simulink model "Ford_T3T6_ArchCnctnDigrm"  (R2016b)
settings: Solver=FixedStepDiscrete  StartTime=0.0  StopTime=10.0  RelTol=1e-3  EnableMultiTasking=on
libraries: canmsglib x15
(part 13 of 15)

== system Ford_T3T6_ArchCnctnDigrm/Vehicle Com/Rx Messages/Vehicle Data ==
  note: From COM
  note: From COM
  note: From COM
  note: From COM
  note: From COM
  Ford_SelDrvMdeChassis2_D_Rq : Ground
  Ignition_Status : Ground
  LifeCycMde_D_Actl : Ground
  MM054A_FordMsg083BusHiSpd : Subsystem  Tag=4.0.X  Description=The purpose of the Ford Message 083 Bus High Speed function is to provide the Electric Power Steering system with signal values for the Lane Detection Warning function from CAN. The Ford Message 083 function will perform the missing message diagnostics as well asprovide a validity flag for the signal values and received message. Detailed requirements have implemented the Ford DBC file for guidance.
      settings: AttributesFormatString=Version: %<Tag>
  MM072A_FordMsg3B3BusHiSpd : Subsystem  Tag=4.0.X  Description=The purpose of the Ford Message 3B3 Bus High Speed function is to provide the Electric PowerSteering system with signal values for the Trailer Back Up Assist and Electric Power Steering functions from CAN. The Ford Message 3B3 function will perform the missing message and signal invalid diagnostic as well as provide a validity signal for the received message.
      settings: AttributesFormatString=Version: %<Tag>
  MM076A_FordMsg40ABusHiSpd : Subsystem  Tag=4.0.X  Description=The purpose of the Ford Message 40A Bus High Speed function is to provide the Electric Power Steering systemwith signal values for the global configuration function from CAN.The Ford Message 40A function will perform the missing message.
      settings: AttributesFormatString=Version: %<Tag>
  MM079A_FordMsg41EBusHiSpd : Subsystem  Tag=4.0.X  Description="The purpose of the Ford Message 41E Bus High Speed function is to providethe Electric Power Steering system with signal values for the Select DriveMode  function from CAN. The Ford Message 41E function will perform themissing message and signal invalid diagnostics as well as provide a validity flag for the signal values and received message."
      settings: AttributesFormatString=Version: %<Tag>
  MM081A_FordMsg430BusHiSpd : Subsystem  Tag=4.0.X  Description=The purpose of the Ford Message 430 Bus High Speed function is to provide the Electric Power Steeringsystem with vehicle odometer, climate, and Trailer Back Up Assist signals from CAN. The Ford Message430 function will perform the missing message and signal invalid diagnostics as well as provide avalidity signal for the signal values and received message.
      settings: AttributesFormatString=Version: %<Tag>
  OdometerMasterValue : Ground
  TurnLghtSwtch_D_Stat : Ground
  VehicleGGCCData : Ground
  tag scope: ComIPduCallout_BodyInfo_3_FD1=global, ComIPduCallout_BrakeSysFeatures_3_FD1=global, ComIPduCallout_Cluster_Info1_FD1=global, ComIPduCallout_GGCC_Config_Mgmt_ID_1_FD1=global, ComIPduCallout_Steering_Data_FD1=global, ComTimeoutNotification_Ignition_Status=global, ComTimeoutNotification_OdometerMasterValue=global, ComTimeoutNotification_SelDrvMdeChassis2_D_Rq=global, ComTimeoutNotification_TurnLghtSwtch_D_Stat=global, ComTimeoutNotification_VehicleGGCCData=global, FordVehGlbRealTi=global, FordVehIdnNr=global, FordVehIgnSts=global, FordVehIgnStsVld=global, FordVehLifeCycMod=global, FordVehOdom=global, FordVehPenSelDrvMod=global, FordVehSelDrvModChassisVld=global, FordVehTireCircum=global, FordVehTurnSigSwtStsRaw=global, FordVehTurnSigVld=global
  wires:
  [ClrDiagcFlgProxy] -> MM054A_FordMsg083BusHiSpd/1(ClrDiagcFlgProxy)
  [FordCanDtcInhb] -> MM054A_FordMsg083BusHiSpd/2(FordCanDtcInhb)
  [FordEpsLifeCycMod] -> MM054A_FordMsg083BusHiSpd/3(FordEpsLifeCycMod)
  [LaneDetnWarnEnad] -> MM054A_FordMsg083BusHiSpd/4(FordLaneDetnWarnEnad)
  TurnLghtSwtch_D_Stat/1 -> MM054A_FordMsg083BusHiSpd/5(Ford_TurnLghtSwtch_D_Stat1)
  [GetRefTmr100MicroSec32bit] -> MM054A_FordMsg083BusHiSpd/6(GetRefTmr100MicroSec32bit)
  [GetTiSpan100MicroSec32bit] -> MM054A_FordMsg083BusHiSpd/7(GetTiSpan100MicroSec32bit)
  [SetNtcSts] -> MM054A_FordMsg083BusHiSpd/8(SetNtcSts)
  MM054A_FordMsg083BusHiSpd/1(FordVehTurnSigSwtStsRaw) -> [FordVehTurnSigSwtStsRaw]
  MM054A_FordMsg083BusHiSpd/2(FordVehTurnSigVld) -> [FordVehTurnSigVld]
  MM054A_FordMsg083BusHiSpd/3(ComIPduCallout_Steering_Data_FD1) -> [ComIPduCallout_Steering_Data_FD1]
  MM054A_FordMsg083BusHiSpd/4(ComTimeoutNotification_TurnLghtSwtch_D_Stat) -> [ComTimeoutNotification_TurnLghtSwtch_D_Stat]
  [ClrDiagcFlgProxy] -> MM072A_FordMsg3B3BusHiSpd/1(ClrDiagcFlgProxy)
  [FordCanDtcInhb] -> MM072A_FordMsg3B3BusHiSpd/2(FordCanDtcInhb)
  [FordEpsLifeCycMod] -> MM072A_FordMsg3B3BusHiSpd/3(FordEpsLifeCycMod)
  Ignition_Status/1 -> MM072A_FordMsg3B3BusHiSpd/4(Ford_Ignition_Status1)
  LifeCycMde_D_Actl/1 -> MM072A_FordMsg3B3BusHiSpd/5(Ford_LifeCycMde_D_Actl1)
  [GetRefTmr100MicroSec32bit] -> MM072A_FordMsg3B3BusHiSpd/6(GetRefTmr100MicroSec32bit)
  [GetTiSpan100MicroSec32bit] -> MM072A_FordMsg3B3BusHiSpd/7(GetTiSpan100MicroSec32bit)
  [SetNtcSts] -> MM072A_FordMsg3B3BusHiSpd/8(SetNtcSts)
  MM072A_FordMsg3B3BusHiSpd/1(FordVehIgnSts) -> [FordVehIgnSts]
  MM072A_FordMsg3B3BusHiSpd/2(FordVehIgnStsVld) -> [FordVehIgnStsVld]
  MM072A_FordMsg3B3BusHiSpd/3(FordVehLifeCycMod) -> [FordVehLifeCycMod]
  MM072A_FordMsg3B3BusHiSpd/4(ComIPduCallout_BodyInfo_3_FD1) -> [ComIPduCallout_BodyInfo_3_FD1]
  MM072A_FordMsg3B3BusHiSpd/5(ComTimeoutNotification_Ignition_Status) -> [ComTimeoutNotification_Ignition_Status]
  [ClrDiagcFlgProxy] -> MM076A_FordMsg40ABusHiSpd/1(ClrDiagcFlgProxy)
  [FordCanDtcInhb] -> MM076A_FordMsg40ABusHiSpd/2(FordCanDtcInhb)
  [FordEpsLifeCycMod] -> MM076A_FordMsg40ABusHiSpd/3(FordEpsLifeCycMod)
  VehicleGGCCData/1 -> MM076A_FordMsg40ABusHiSpd/4(Ford_VehicleGGCCData)
  [GetRefTmr100MicroSec32bit] -> MM076A_FordMsg40ABusHiSpd/5(GetRefTmr100MicroSec32bit)
  [GetTiSpan100MicroSec32bit] -> MM076A_FordMsg40ABusHiSpd/6(GetTiSpan100MicroSec32bit)
  [SetNtcSts] -> MM076A_FordMsg40ABusHiSpd/7(SetNtcSts)
  MM076A_FordMsg40ABusHiSpd/1(FordVehGlbRealTi) -> [FordVehGlbRealTi]
  MM076A_FordMsg40ABusHiSpd/2(FordVehIdnNr) -> [FordVehIdnNr]
  MM076A_FordMsg40ABusHiSpd/3(FordVehTireCircum) -> [FordVehTireCircum]
  MM076A_FordMsg40ABusHiSpd/4(ComIPduCallout_GGCC_Config_Mgmt_ID_1_FD1) -> [ComIPduCallout_GGCC_Config_Mgmt_ID_1_FD1]
  MM076A_FordMsg40ABusHiSpd/5(ComTimeoutNotification_VehicleGGCCData) -> [ComTimeoutNotification_VehicleGGCCData]
  [ClrDiagcFlgProxy] -> MM081A_FordMsg430BusHiSpd/1(ClrDiagcFlgProxy)
  [FordCanDtcInhb] -> MM081A_FordMsg430BusHiSpd/2(FordCanDtcInhb)
  [FordEpsLifeCycMod] -> MM081A_FordMsg430BusHiSpd/3(FordEpsLifeCycMod)
  OdometerMasterValue/1 -> MM081A_FordMsg430BusHiSpd/4(Ford_OdometerMasterValue)
  [GetRefTmr100MicroSec32bit] -> MM081A_FordMsg430BusHiSpd/5(GetRefTmr100MicroSec32bit)
  [GetTiSpan100MicroSec32bit] -> MM081A_FordMsg430BusHiSpd/6(GetTiSpan100MicroSec32bit)
  [SetNtcSts] -> MM081A_FordMsg430BusHiSpd/7(SetNtcSts)
  MM081A_FordMsg430BusHiSpd/1(FordVehOdom) -> [FordVehOdom]
  MM081A_FordMsg430BusHiSpd/2(ComIPduCallout_Cluster_Info1_FD1) -> [ComIPduCallout_Cluster_Info1_FD1]
  MM081A_FordMsg430BusHiSpd/3(ComTimeoutNotification_OdometerMasterValue) -> [ComTimeoutNotification_OdometerMasterValue]
  [ClrDiagcFlgProxy] -> MM079A_FordMsg41EBusHiSpd/1(ClrDiagcFlgProxy)
  [FordCanDtcInhb] -> MM079A_FordMsg41EBusHiSpd/2(FordCanDtcInhb)
  [FordEpsLifeCycMod] -> MM079A_FordMsg41EBusHiSpd/3(FordEpsLifeCycMod)
  [FordSelDrvModEnad] -> MM079A_FordMsg41EBusHiSpd/4(FordSelDrvModEnad)
  Ford_SelDrvMdeChassis2_D_Rq/1 -> MM079A_FordMsg41EBusHiSpd/5(Ford_SelDrvMdeChassis2_D_Rq1)
  [GetRefTmr100MicroSec32bit] -> MM079A_FordMsg41EBusHiSpd/6(GetRefTmr100MicroSec32bit)
  [GetTiSpan100MicroSec32bit] -> MM079A_FordMsg41EBusHiSpd/7(GetTiSpan100MicroSec32bit)
  [SetNtcSts] -> MM079A_FordMsg41EBusHiSpd/8(SetNtcSts)
  MM079A_FordMsg41EBusHiSpd/1(FordVehPenSelDrvMod) -> [FordVehPenSelDrvMod]
  MM079A_FordMsg41EBusHiSpd/2(FordVehSelDrvModChassisVld) -> [FordVehSelDrvModChassisVld]
  MM079A_FordMsg41EBusHiSpd/3(ComIPduCallout_BrakeSysFeatures_3_FD1) -> [ComIPduCallout_BrakeSysFeatures_3_FD1]
  MM079A_FordMsg41EBusHiSpd/4(ComTimeoutNotification_SelDrvMdeChassis2_D_Rq) -> [ComTimeoutNotification_SelDrvMdeChassis2_D_Rq]

== system Ford_T3T6_ArchCnctnDigrm/Vehicle Com/Rx Messages/Wheel Data ==
  note: From COM
  note: From COM
  note: From COM
  note: From COM
  ElPw_D_Stat : Ground
  ElPw_D_StatStrtStop : Ground
  Ground : Ground
  MM055A_FordMsg08ABusHiSpd : Subsystem  Tag=4.0.X  Description=The purpose of the Ford Message 08A Bus High Speed function is to provide the Electric Power Steering system with signal values for the EAC feature. The Ford Message 08A function will perform the missing message and signal invalid diagnostics
      settings: AttributesFormatString=Version: %<Tag>
  MM059A_FordMsg167BusHiSpd : Subsystem  Tag=2.0.0  Description=The purpose of the Ford Message 0167 Bus HighSpeed function is to provide the EPS system with signal valuesfor the System State, Voltage Diagnostic, Start Stop, and TorqueSteer Compensation functions from CAN. The Ford Message 167 functionwill perform the missing message and signal invalid diagnostics aswell as provide a validity flag for the signal valuesand received message.
      settings: AttributesFormatString=Version: %<Tag>
  MM064A_FordMsg216BusHiSpd : Subsystem  Tag=4.0.X  Description=The purpose of the Ford Message 216 Bus High Speedfunction is to provide the Electric Power Steering system with signalvalues for the Trailer Back Up Assist, Torque Steer Compensation,and Brake Oscillation Reduction functions from CAN. The Ford Message216 function will perform the missing message diagnostic as wellas provide a validity signal for the received message.
      settings: AttributesFormatString=Version: %<Tag>
  MM065A_FordMsg217BusHiSpd : Subsystem  Tag=4.0.X  Description=The purpose of the Ford Message 217 Bus High Speed function is to providethe Electric Power Steering system with signal values for vehicle speed, Active Nibble Control,TSC, Brake Oscillation Reduction, and Trailer Back Up Assist functions from CAN. The Ford Message 217Bus High Speed function will perform the missing message and signal invalid diagnostics as well as providea validity signal for the signal values and received message.
      settings: AttributesFormatString=Version: %<Tag>
  PrplWhlTot2_Tq_Actl : Ground
  PwPckTq_D_Stat : Ground
  SteWhlRelCalib_An_Sns1 : Ground
  WhlFl_W_Meas1 : Ground
  WhlFr_W_Meas1 : Ground
  WhlRl_W_Meas1 : Ground
  WhlRr_W_Meas1 : Ground
  tag scope: ComIPduCallout_ActiveFrontSteering_Stat2_FD1=global, ComIPduCallout_VehicleOperatingModes_HS2=global, ComIPduCallout_WheelData_FD1=global, ComIPduCallout_WheelSpeed_FD1=global, ComTimeoutNotification_PwPckTq_D_Stat=global, ComTimeoutNotification_SteWhlRelCalib_An_Sns=global, ComTimeoutNotification_WhlDirFl_D_Actl=global, ComTimeoutNotification_WhlFl_W_Meas=global, FordActvFrntSteerModlSteerWhlAgVldInt=global, FordVehActvFrntSteerModlSteerWhlAg=global, FordVehActvFrntSteerModlSteerWhlAgRaw=global, FordVehElecPwrStrtStopSts=global, FordVehElecPwrSts=global, FordVehFrntLeWhlCntrDirVld=global, FordVehFrntLeWhlDirRaw=global, FordVehFrntLeWhlRollgCntr=global, FordVehFrntLeWhlSpd=global, FordVehFrntLeWhlSpdRaw=global, FordVehFrntLeWhlSpdVld=global, FordVehFrntRiWhlCntrDirVld=global, FordVehFrntRiWhlDirRaw=global, FordVehFrntRiWhlRollgCntr=global, FordVehFrntRiWhlSpd=global, FordVehFrntRiWhlSpdRaw=global, FordVehFrntRiWhlSpdVld=global, FordVehPrpnWhlTq=global, FordVehPrpnWhlTqRaw=global, FordVehPrpnWhlTqVld=global, FordVehPwrpkTqSts=global, FordVehReLeWhlCntrDirVld=global, FordVehReLeWhlDirRaw=global, FordVehReLeWhlRollgCntr=global, FordVehReLeWhlSpd=global, FordVehReLeWhlSpdRaw=global, FordVehReLeWhlSpdVld=global, FordVehReRiWhlCntrDirVld=global, FordVehReRiWhlDirRaw=global, FordVehReRiWhlRollgCntr=global, FordVehReRiWhlSpd=global, FordVehReRiWhlSpdRaw=global, FordVehReRiWhlSpdVld=global
  wires:
  [ClrDiagcFlgProxy] -> MM059A_FordMsg167BusHiSpd/1(ClrDiagcFlgProxy)
  [FordBrkOscnRednEnad] -> MM059A_FordMsg167BusHiSpd/2(FordBrkOscnRednEnad)
  [FordCanDtcInhb] -> MM059A_FordMsg167BusHiSpd/3(FordCanDtcInhb)
  [FordEpsLifeCycMod] -> MM059A_FordMsg167BusHiSpd/4(FordEpsLifeCycMod)
  [FordInvldMsgDiagcInhb] -> MM059A_FordMsg167BusHiSpd/5(FordInvldMsgDiagcInhb)
  [FordMfgDiagcInhb] -> MM059A_FordMsg167BusHiSpd/6(FordMfgDiagcInhb)
  [FordMissMsgDiagcInhb] -> MM059A_FordMsg167BusHiSpd/7(FordMissMsgDiagcInhb)
  [FordTqSteerCmpEnad] -> MM059A_FordMsg167BusHiSpd/8(FordTqSteerCmpEnad)
  [FordTrlrBackupAssiEnad] -> MM059A_FordMsg167BusHiSpd/9(FordTrlrBackUpAssiEnad)
  ElPw_D_Stat/1 -> MM059A_FordMsg167BusHiSpd/10(Ford_ElPw_D_Stat1)
  [GetRefTmr100MicroSec32bit] -> MM059A_FordMsg167BusHiSpd/14(GetRefTmr100MicroSec32bit)
  [GetTiSpan100MicroSec32bit] -> MM059A_FordMsg167BusHiSpd/15(GetTiSpan100MicroSec32bit)
  [SetNtcSts] -> MM059A_FordMsg167BusHiSpd/16(SetNtcSts)
  MM059A_FordMsg167BusHiSpd/1(FordVehElecPwrStrtStopSts) -> [FordVehElecPwrStrtStopSts]
  MM059A_FordMsg167BusHiSpd/2(FordVehElecPwrSts) -> [FordVehElecPwrSts]
  MM059A_FordMsg167BusHiSpd/3(FordVehPrpnWhlTq) -> [FordVehPrpnWhlTq]
  MM059A_FordMsg167BusHiSpd/4(FordVehPrpnWhlTqRaw) -> [FordVehPrpnWhlTqRaw]
  MM059A_FordMsg167BusHiSpd/5(FordVehPrpnWhlTqVld) -> [FordVehPrpnWhlTqVld]
  MM059A_FordMsg167BusHiSpd/6(FordVehPwrpkTqSts) -> [FordVehPwrpkTqSts]
  MM059A_FordMsg167BusHiSpd/7(ComIPduCallout_VehicleOperatingModes_HS2) -> [ComIPduCallout_VehicleOperatingModes_HS2]
  MM059A_FordMsg167BusHiSpd/8(ComTimeoutNotification_PwPckTq_D_Stat) -> [ComTimeoutNotification_PwPckTq_D_Stat]
  ElPw_D_StatStrtStop/1 -> MM059A_FordMsg167BusHiSpd/11(Ford_ElPw_D_StatStrtStop1)
  PrplWhlTot2_Tq_Actl/1 -> MM059A_FordMsg167BusHiSpd/12(Ford_PrplWhlTot2_Tq_Actl)
  PwPckTq_D_Stat/1 -> MM059A_FordMsg167BusHiSpd/13(Ford_PwPckTq_D_Stat1)
  [ClrDiagcFlgProxy] -> MM065A_FordMsg217BusHiSpd/1(ClrDiagcFlgProxy)
  [FordAbsPrsnt] -> MM065A_FordMsg217BusHiSpd/2(FordAbsPrsnt)
  [FordActvNiblCtrlEnad] -> MM065A_FordMsg217BusHiSpd/3(FordActvNiblCtrlEnad)
  [FordBrkOscnRednEnad] -> MM065A_FordMsg217BusHiSpd/4(FordBrkOscnRednEnad)
  [FordCanDtcInhb] -> MM065A_FordMsg217BusHiSpd/5(FordCanDtcInhb)
  [FordEpsLifeCycMod] -> MM065A_FordMsg217BusHiSpd/6(FordEpsLifeCycMod)
  [FordTqSteerCmpEnad] -> MM065A_FordMsg217BusHiSpd/7(FordTqSteerCmpEnad)
  [FordTrlrBackupAssiEnad] -> MM065A_FordMsg217BusHiSpd/8(FordTrlrBackupAssiEnad)
  [GetRefTmr100MicroSec32bit] -> MM065A_FordMsg217BusHiSpd/13(GetRefTmr100MicroSec32bit)
  [GetTiSpan100MicroSec32bit] -> MM065A_FordMsg217BusHiSpd/14(GetTiSpan100MicroSec32bit)
  [SetNtcSts] -> MM065A_FordMsg217BusHiSpd/15(SetNtcSts)
  MM065A_FordMsg217BusHiSpd/1(FordVehFrntLeWhlSpd) -> [FordVehFrntLeWhlSpd]
  MM065A_FordMsg217BusHiSpd/2(FordVehFrntLeWhlSpdRaw) -> [FordVehFrntLeWhlSpdRaw]
  MM065A_FordMsg217BusHiSpd/3(FordVehFrntLeWhlSpdVld) -> [FordVehFrntLeWhlSpdVld]
  MM065A_FordMsg217BusHiSpd/4(FordVehFrntRiWhlSpd) -> [FordVehFrntRiWhlSpd]
  MM065A_FordMsg217BusHiSpd/5(FordVehFrntRiWhlSpdRaw) -> [FordVehFrntRiWhlSpdRaw]
  MM065A_FordMsg217BusHiSpd/6(FordVehFrntRiWhlSpdVld) -> [FordVehFrntRiWhlSpdVld]
  MM065A_FordMsg217BusHiSpd/7(FordVehReLeWhlSpd) -> [FordVehReLeWhlSpd]
  MM065A_FordMsg217BusHiSpd/8(FordVehReLeWhlSpdRaw) -> [FordVehReLeWhlSpdRaw]
  MM065A_FordMsg217BusHiSpd/9(FordVehReLeWhlSpdVld) -> [FordVehReLeWhlSpdVld]
  MM065A_FordMsg217BusHiSpd/10(FordVehReRiWhlSpd) -> [FordVehReRiWhlSpd]
  MM065A_FordMsg217BusHiSpd/11(FordVehReRiWhlSpdRaw) -> [FordVehReRiWhlSpdRaw]
  MM065A_FordMsg217BusHiSpd/12(FordVehReRiWhlSpdVld) -> [FordVehReRiWhlSpdVld]
  MM065A_FordMsg217BusHiSpd/13(ComIPduCallout_WheelSpeed_FD1) -> [ComIPduCallout_WheelSpeed_FD1]
  MM065A_FordMsg217BusHiSpd/14(ComTimeoutNotification_WhlFl_W_Meas) -> [ComTimeoutNotification_WhlFl_W_Meas]
  WhlFl_W_Meas1/1 -> MM065A_FordMsg217BusHiSpd/9(Ford_WhlFl_W_Meas)
  WhlFr_W_Meas1/1 -> MM065A_FordMsg217BusHiSpd/10(Ford_WhlFr_W_Meas)
  WhlRl_W_Meas1/1 -> MM065A_FordMsg217BusHiSpd/11(Ford_WhlRl_W_Meas)
  WhlRr_W_Meas1/1 -> MM065A_FordMsg217BusHiSpd/12(Ford_WhlRr_W_Meas)
  [ClrDiagcFlgProxy] -> MM064A_FordMsg216BusHiSpd/1(ClrDiagcFlgProxy)
  [FordBrkOscnRednEnad] -> MM064A_FordMsg216BusHiSpd/2(FordBrkOscnRednEnad)
  [FordCanDtcInhb] -> MM064A_FordMsg216BusHiSpd/3(FordCanDtcInhb)
  [FordEpsLifeCycMod] -> MM064A_FordMsg216BusHiSpd/4(FordEpsLifeCycMod)
  [FordMfgDiagcInhb] -> MM064A_FordMsg216BusHiSpd/5(FordMfgDiagcInhb)
  [FordMissMsgDiagcInhb] -> MM064A_FordMsg216BusHiSpd/6(FordMissMsgDiagcInhb)
  [FordTqSteerCmpEnad] -> MM064A_FordMsg216BusHiSpd/7(FordTqSteerCmpEnad)
  [FordTrlrBackupAssiEnad] -> MM064A_FordMsg216BusHiSpd/8(FordTrlrBackUpAssiEnad)
  Ground/1 -> MM064A_FordMsg216BusHiSpd/16(Ford_WhlRotatRr_No_Cnt), MM064A_FordMsg216BusHiSpd/15(Ford_WhlRotatRl_No_Cnt), MM064A_FordMsg216BusHiSpd/14(Ford_WhlRotatFr_No_Cnt), MM064A_FordMsg216BusHiSpd/13(Ford_WhlRotatFl_No_Cnt), MM064A_FordMsg216BusHiSpd/12(Ford_WhlDirRr_D_Actl1), MM064A_FordMsg216BusHiSpd/11(Ford_WhlDirRl_D_Actl1), MM064A_FordMsg216BusHiSpd/10(Ford_WhlDirFr_D_Actl1), MM064A_FordMsg216BusHiSpd/9(Ford_WhlDirFl_D_Actl1)
  [GetRefTmr100MicroSec32bit] -> MM064A_FordMsg216BusHiSpd/17(GetRefTmr100MicroSec32bit)
  [GetTiSpan100MicroSec32bit] -> MM064A_FordMsg216BusHiSpd/18(GetTiSpan100MicroSec32bit)
  [SetNtcSts] -> MM064A_FordMsg216BusHiSpd/19(SetNtcSts)
  MM064A_FordMsg216BusHiSpd/1(FordVehFrntLeWhlCntrDirVld) -> [FordVehFrntLeWhlCntrDirVld]
  MM064A_FordMsg216BusHiSpd/2(FordVehFrntLeWhlDirRaw) -> [FordVehFrntLeWhlDirRaw]
  MM064A_FordMsg216BusHiSpd/3(FordVehFrntLeWhlRollgCntr) -> [FordVehFrntLeWhlRollgCntr]
  MM064A_FordMsg216BusHiSpd/4(FordVehFrntRiWhlCntrDirVld) -> [FordVehFrntRiWhlCntrDirVld]
  MM064A_FordMsg216BusHiSpd/5(FordVehFrntRiWhlDirRaw) -> [FordVehFrntRiWhlDirRaw]
  MM064A_FordMsg216BusHiSpd/6(FordVehFrntRiWhlRollgCntr) -> [FordVehFrntRiWhlRollgCntr]
  MM064A_FordMsg216BusHiSpd/7(FordVehReLeWhlCntrDirVld) -> [FordVehReLeWhlCntrDirVld]
  MM064A_FordMsg216BusHiSpd/8(FordVehReLeWhlDirRaw) -> [FordVehReLeWhlDirRaw]
  MM064A_FordMsg216BusHiSpd/9(FordVehReLeWhlRollgCntr) -> [FordVehReLeWhlRollgCntr]
  MM064A_FordMsg216BusHiSpd/10(FordVehReRiWhlCntrDirVld) -> [FordVehReRiWhlCntrDirVld]
  MM064A_FordMsg216BusHiSpd/11(FordVehReRiWhlDirRaw) -> [FordVehReRiWhlDirRaw]
  MM064A_FordMsg216BusHiSpd/12(FordVehReRiWhlRollgCntr) -> [FordVehReRiWhlRollgCntr]
  MM064A_FordMsg216BusHiSpd/13(ComIPduCallout_WheelData_FD1) -> [ComIPduCallout_WheelData_FD1]
  MM064A_FordMsg216BusHiSpd/14(ComTimeoutNotification_WhlDirFl_D_Actl) -> [ComTimeoutNotification_WhlDirFl_D_Actl]
  [ClrDiagcFlgProxy] -> MM055A_FordMsg08ABusHiSpd/1(ClrDiagcFlgProxy)
  [ActvFrntSteerPrsnt] -> MM055A_FordMsg08ABusHiSpd/2(FordActvFrntSteerPrsnt)
  [FordCanDtcInhb] -> MM055A_FordMsg08ABusHiSpd/3(FordCanDtcInhb)
  [FordEpsLifeCycMod] -> MM055A_FordMsg08ABusHiSpd/4(FordEpsLifeCycMod)
  SteWhlRelCalib_An_Sns1/1 -> MM055A_FordMsg08ABusHiSpd/5(Ford_SteWhlRelCalib_An_Sns)
  [GetRefTmr100MicroSec32bit] -> MM055A_FordMsg08ABusHiSpd/6(GetRefTmr100MicroSec32bit)
  [GetTiSpan100MicroSec32bit] -> MM055A_FordMsg08ABusHiSpd/7(GetTiSpan100MicroSec32bit)
  [SetNtcSts] -> MM055A_FordMsg08ABusHiSpd/8(SetNtcSts)
  MM055A_FordMsg08ABusHiSpd/1(FordActvFrntSteerModlSteerWhlAgVldInt) -> [FordActvFrntSteerModlSteerWhlAgVldInt]
  MM055A_FordMsg08ABusHiSpd/2(FordVehActvFrntSteerModlSteerWhlAg) -> [FordVehActvFrntSteerModlSteerWhlAg]
  MM055A_FordMsg08ABusHiSpd/3(FordVehActvFrntSteerModlSteerWhlAgRaw) -> [FordVehActvFrntSteerModlSteerWhlAgRaw]
  MM055A_FordMsg08ABusHiSpd/4(ComIPduCallout_ActiveFrontSteering_Stat2_FD1) -> [ComIPduCallout_ActiveFrontSteering_Stat2_FD1]
  MM055A_FordMsg08ABusHiSpd/5(ComTimeoutNotification_SteWhlRelCalib_An_Sns) -> [ComTimeoutNotification_SteWhlRelCalib_An_Sns]

== system Ford_T3T6_ArchCnctnDigrm/Vehicle Com/Rx Messages/Yaw Rate ==
  note: From COM
  note: From COM
  note: From COM
  Ford_TrlrSnsId_No_Act : Ground
  MM056A_FordMsg091BusHiSpd : Subsystem  Tag=0.0.X
      settings: AttributesFormatString=Version: %<Tag>
  MM082A_FordMsg452BusHiSpd : Subsystem  Tag=1.0.X  Description=The purpose of the Ford Message 452 Bus High Speed function is to provide the Electric Power Steering system with Trailer Back up Assist and Gear Lever Position signals from CAN. The Ford Message 452 function will perform the missing message and signal invalid diagnostics as well as provide a validity signal for the signal values and received message.
      settings: AttributesFormatString=Version: %<Tag>
  MM089A_FordMsg4B0BusHiSpd : Subsystem  Tag=4.0.X  Description=The purpose of the Ford Message 4B0 Bus High Speed function is to provide the Electric Power Steering system with signal values for the Torque Steer Compensation, Brake Oscillation Reduction, Lane Detection Warning, LKA, Traffic Jam Assist, Lane Center Assist, and Evasive Steer Assist functions from CAN. The Ford Message 4B0 function will perform the missing message and signal invalid diagnostics as well as provide a validity flag for the signal values and received message.
      settings: AttributesFormatString=Version: %<Tag>
  VehYaw_W_Actl : Ground
  YawStabilityIndex : Ground
  tag scope: ComIPduCallout_ABS_BrkBst_Data_FD1=global, ComIPduCallout_TrailerAid_Stat1_FD1=global, ComIPduCallout_Yaw_Data_FD1=global, ComTimeoutNotification_TrlrSnsId_No_Actl=global, ComTimeoutNotification_VehYaw_W_Actl=global, ComTimeoutNotification_YawStabilityIndex=global, FordVehYawRate=global, FordVehYawRateRaw=global, FordVehYawRateRawVld=global, FordVehYawRateSnsrIdyHi=global, FordVehYawRateSnsrIdyLo=global, FordVehYawStabyRaw=global, FordVehYawStabyVld=global
  wires:
  [ClrDiagcFlgProxy] -> MM056A_FordMsg091BusHiSpd/1(ClrDiagcFlgProxy)
  [FordCanDtcInhb] -> MM056A_FordMsg091BusHiSpd/2(FordCanDtcInhb)
  [FordEpsLifeCycMod] -> MM056A_FordMsg091BusHiSpd/3(FordEpsLifeCycMod)
  [FordInvldMsgDiagcInhb] -> MM056A_FordMsg091BusHiSpd/4(FordInvldMsgDiagcInhb)
  [FordMfgDiagcInhb] -> MM056A_FordMsg091BusHiSpd/5(FordMfgDiagcInhb)
  [FordMissMsgDiagcInhb] -> MM056A_FordMsg091BusHiSpd/6(FordMissMsgDiagcInhb)
  [FordTrlrBackupAssiEnad] -> MM056A_FordMsg091BusHiSpd/7(FordTrlrBackupAssiEnad)
  VehYaw_W_Actl/1 -> MM056A_FordMsg091BusHiSpd/8(Ford_VehYaw_W_Actl)
  [FordLaneCentrAssiEnad] -> MM056A_FordMsg091BusHiSpd/9(FordLaneCentrAssiEnad)
  [FordTrfcJamAssiEnad] -> MM056A_FordMsg091BusHiSpd/10(FordTrfcJamAssiEnad)
  [GetRefTmr100MicroSec32bit] -> MM056A_FordMsg091BusHiSpd/11(GetRefTmr100MicroSec32bit)
  [GetTiSpan100MicroSec32bit] -> MM056A_FordMsg091BusHiSpd/12(GetTiSpan100MicroSec32bit)
  [SetNtcSts] -> MM056A_FordMsg091BusHiSpd/13(SetNtcSts)
  MM056A_FordMsg091BusHiSpd/1(FordVehYawRate) -> [FordVehYawRate]
  MM056A_FordMsg091BusHiSpd/2(FordVehYawRateRaw) -> [FordVehYawRateRaw]
  MM056A_FordMsg091BusHiSpd/3(FordVehYawRateRawVld) -> [FordVehYawRateRawVld]
  MM056A_FordMsg091BusHiSpd/4(ComIPduCallout_Yaw_Data_FD1) -> [ComIPduCallout_Yaw_Data_FD1]
  MM056A_FordMsg091BusHiSpd/5(ComTimeoutNotification_VehYaw_W_Actl) -> [ComTimeoutNotification_VehYaw_W_Actl]
  [ClrDiagcFlgProxy] -> MM082A_FordMsg452BusHiSpd/1(ClrDiagcFlgProxy)
  [FordCanDtcInhb] -> MM082A_FordMsg452BusHiSpd/2(FordCanDtcInhb)
  [FordEpsLifeCycMod] -> MM082A_FordMsg452BusHiSpd/3(FordEpsLifeCycMod)
  [FordInvldMsgDiagcInhb] -> MM082A_FordMsg452BusHiSpd/4(FordInvldMsgDiagcInhb)
  [FordMfgDiagcInhb] -> MM082A_FordMsg452BusHiSpd/5(FordMfgDiagcInhb)
  [FordMissMsgDiagcInhb] -> MM082A_FordMsg452BusHiSpd/6(FordMissMsgDiagcInhb)
  [FordTrlrBackupAssiEnad] -> MM082A_FordMsg452BusHiSpd/7(FordTrlrBackupAssiEnad)
  Ford_TrlrSnsId_No_Act/1 -> MM082A_FordMsg452BusHiSpd/8(Ford_TrlrSnsId_No_Act)
  [GetRefTmr100MicroSec32bit] -> MM082A_FordMsg452BusHiSpd/9(GetRefTmr100MicroSec32bit)
  [GetTiSpan100MicroSec32bit] -> MM082A_FordMsg452BusHiSpd/10(GetTiSpan100MicroSec32bit)
  [SetNtcSts] -> MM082A_FordMsg452BusHiSpd/11(SetNtcSts)
  MM082A_FordMsg452BusHiSpd/1(FordVehYawRateSnsrIdyHi) -> [FordVehYawRateSnsrIdyHi]
  MM082A_FordMsg452BusHiSpd/2(FordVehYawRateSnsrIdyLo) -> [FordVehYawRateSnsrIdyLo]
  MM082A_FordMsg452BusHiSpd/3(ComIPduCallout_TrailerAid_Stat1_FD1) -> [ComIPduCallout_TrailerAid_Stat1_FD1]
  MM082A_FordMsg452BusHiSpd/4(ComTimeoutNotification_TrlrSnsId_No_Actl) -> [ComTimeoutNotification_TrlrSnsId_No_Actl]
  [ClrDiagcFlgProxy] -> MM089A_FordMsg4B0BusHiSpd/1(ClrDiagcFlgProxy)
  [FordBrkOscnRednEnad] -> MM089A_FordMsg4B0BusHiSpd/2(FordBrkOscnRednEnad)
  [FordCanDtcInhb] -> MM089A_FordMsg4B0BusHiSpd/3(FordCanDtcInhb)
  [FordEpsLifeCycMod] -> MM089A_FordMsg4B0BusHiSpd/4(FordEpsLifeCycMod)
  [FordEvasSteerAssiEnad] -> MM089A_FordMsg4B0BusHiSpd/5(FordEvasSteerAssiEnad)
  [FordInvldMsgDiagcInhb] -> MM089A_FordMsg4B0BusHiSpd/6(FordInvldMsgDiagcInhb)
  [FordLaneCentrAssiEnad] -> MM089A_FordMsg4B0BusHiSpd/7(FordLaneCentrAssiEnad)
  [FordMfgDiagcInhb] -> MM089A_FordMsg4B0BusHiSpd/8(FordMfgDiagcInhb)
  [FordMissMsgDiagcInhb] -> MM089A_FordMsg4B0BusHiSpd/9(FordMissMsgDiagcInhb)
  [FordTqSteerCmpEnad] -> MM089A_FordMsg4B0BusHiSpd/10(FordTqSteerCmpEnad)
  YawStabilityIndex/1 -> MM089A_FordMsg4B0BusHiSpd/11(Ford_YawStabilityIndex)
  [LaneDetnWarnEnad] -> MM089A_FordMsg4B0BusHiSpd/12(LaneDetnWarnEnad)
  [FordLaneKeepAssiEnad] -> MM089A_FordMsg4B0BusHiSpd/13(LaneKeepAssiEnad)
  [FordTrfcJamAssiEnad] -> MM089A_FordMsg4B0BusHiSpd/14(TrfcJamAssiEnad)
  [GetRefTmr100MicroSec32bit] -> MM089A_FordMsg4B0BusHiSpd/15(GetRefTmr100MicroSec32bit)
  [GetTiSpan100MicroSec32bit] -> MM089A_FordMsg4B0BusHiSpd/16(GetTiSpan100MicroSec32bit)
  [SetNtcSts] -> MM089A_FordMsg4B0BusHiSpd/17(SetNtcSts)
  MM089A_FordMsg4B0BusHiSpd/1(FordVehYawStabyRaw) -> [FordVehYawStabyRaw]
  MM089A_FordMsg4B0BusHiSpd/2(FordVehYawStabyVld) -> [FordVehYawStabyVld]
  MM089A_FordMsg4B0BusHiSpd/3(ComIPduCallout_ABS_BrkBst_Data_FD1) -> [ComIPduCallout_ABS_BrkBst_Data_FD1]
  MM089A_FordMsg4B0BusHiSpd/4(ComTimeoutNotification_YawStabilityIndex) -> [ComTimeoutNotification_YawStabilityIndex]

== system Ford_T3T6_ArchCnctnDigrm/Vehicle Com/Tx Messages/MM518A_FordMsg417BusHiSpd ==
  FordVehEvasSteerAssiSts : Inport
  FordVehLatCtrlLimSts : Inport  Port=2
  FordVehLatCtrlSteerSts : Inport  Port=3
  FordVehSelDrvModSteerSts : Inport  Port=4
  FordVehTrlrAidAgMax : Inport  Port=5
  FordVehTrlrAidAgOffs : Inport  Port=6
  FordVehTrlrAidAgWarn : Inport  Port=7
  FordVehTrlrAidEnaSts : Inport  Port=8
  FordVehTrlrAidHitchToAxle : Inport  Port=9
  FordVehTrlrAidMsgTxtReq : Inport  Port=10
  FordVehTrlrAidSetUp : Inport  Port=11
  FordVehTrlrAidTarIdn : Inport  Port=12
  FordVehTrlrAidTrlrIdn : Inport  Port=13
  Ford_EsaOn_B_Stat1 : Outport
  Ford_HitchToTrlrAxle_L_Calc : Outport  Port=2
  Ford_LatCtlLim_D_Stat1 : Outport  Port=3
  Ford_LatCtlSte_D_Stat1 : Outport  Port=4
  Ford_SelDrvMdeSte_D_Stat1 : Outport  Port=5
  Ford_TrlrAidEnbl_D2_Stat1 : Outport  Port=6
  Ford_TrlrAidMsgTxt_D2_Rq1 : Outport  Port=7
  Ford_TrlrAidSetup_D2_Stat1 : Outport  Port=8
  Ford_TrlrAidTrgtId_No_Rq : Outport  Port=9
  Ford_TrlrAidTrlrId_No_Rq : Outport  Port=10
  Ford_TrlrAnOffst_An2_Calc : Outport  Port=11
  Ford_TrlrAn_An_MxCalc : Outport  Port=12
  Ford_TrlrAn_An_WarnCalc : Outport  Port=13

== system Ford_T3T6_ArchCnctnDigrm/Vehicle Com/Tx Messages/MM519A_FordMsg5B5BusHiSpd ==
  PSCM_AutoSarNMControl : Outport
  PSCM_AutoSarNMNodeId : Outport  Port=2
  PSCM_AutoSarNMReserved1 : Outport  Port=3
  PSCM_AutoSarNMReserved2 : Outport  Port=4
  PSCM_AutoSarNMReserved3 : Outport  Port=5
  PSCM_AutoSarNMReserved4 : Outport  Port=6
  PSCM_GWNMProxy : Outport  Port=7
  PSCM_GWOnBoardTester : Outport  Port=8

== system Ford_T3T6_ArchCnctnDigrm/Vehicle Com/Tx Messages/MM531A_FordMsg07EBusHiSpd ==
  CmpdSteerPinionAg : Inport
  CmpdSteerPinionAgQlyFac : Inport  Port=2
  FordVehSteerPwrReq : Inport  Port=3
  RelSteerPinionAg : Inport  Port=4
  Ford_StePinAn_No_Cnt : Outport
  Ford_StePinAn_No_Cs : Outport  Port=2
  Ford_StePinCompAnEst_D_Qf1 : Outport  Port=3
  Ford_StePinComp_An_Est : Outport  Port=4
  Ford_StePinRelInit_An_Sns : Outport  Port=5
  Ford_StePw_B_Rq1 : Outport  Port=6

== system Ford_T3T6_ArchCnctnDigrm/Vehicle Com/Tx Messages/MM532A_FordMsg082BusHiSpd ==
  ElecPwrSteerCurr : Inport
  ElecPwrSteerVltg : Inport  Port=2
  FordElecPwrAssidSteerFailr : Inport  Port=3
  FordSteerModlSts : Inport  Port=4
  FordVehDrvrSteerActvnSts : Inport  Port=5
  FordVehDrvrSteerTqReq : Inport  Port=6
  FordVehReCamrLiSts : Inport  Port=7
  FordVehSAPPAgCtrlSts1 : Inport  Port=8
  FordVehSAPPAgCtrlSts2 : Inport  Port=9
  FordVehSAPPAgCtrlSts3 : Inport  Port=10
  FordVehSAPPAgCtrlSts4 : Inport  Port=11
  FordVehSAPPAgCtrlSts5 : Inport  Port=12
  FordVehSAPPAgCtrlSts6 : Inport  Port=13
  FordVehVelMaxReqTrlrAid : Inport  Port=14
  FordVehVelTrlrAidReq : Inport  Port=15
  InpTqRaw : Inport  Port=16
  Ford_DrvSteActv_B_Stat1 : Outport
  Ford_DrvSte_Tq_Actl : Outport  Port=2
  Ford_EPAS_Failure1 : Outport  Port=3
  Ford_SAPPAngleControlStat1_1 : Outport  Port=4
  Ford_SAPPAngleControlStat2_1 : Outport  Port=5
  Ford_SAPPAngleControlStat3_1 : Outport  Port=6
  Ford_SAPPAngleControlStat4_1 : Outport  Port=7
  Ford_SAPPAngleControlStat5_1 : Outport  Port=8
  Ford_SAPPAngleControlStat6_1 : Outport  Port=9
  Ford_SteMdule_D_Stat1 : Outport  Port=10
  Ford_SteMdule_I_Est : Outport  Port=11
  Ford_SteMdule_U_Meas : Outport  Port=12
  Ford_SteeringColumnTorque : Outport  Port=13
  Ford_TrlrHitchLamp_D_Rqst1 : Outport  Port=14
  Ford_VehVTrlrAid_B_Rq1 : Outport  Port=15
  Ford_Veh_V_RqMxTrlrAid : Outport  Port=16

== system Ford_T3T6_ArchCnctnDigrm/Vehicle Com/Tx Messages/MM533A_FordMsg3CCBusHiSpd ==
  FordVehLaneAssiAvl : Inport
  FordVehLaneAssiHandsOff : Inport  Port=2
  FordVehLaneAssiRejctn : Inport  Port=3
  FordVehLoSpdMtnCtrlBrkDecelEna : Inport  Port=4
  FordVehLoSpdMtnCtrlBrkTqReq : Inport  Port=5
  FordVehTrfcJamAvdHandsOnConf : Inport  Port=6
  FordVehTrlrAgTarCalcn : Inport  Port=7
  Ford_LaActAvail_D_Actl1 : Outport
  Ford_LaActDeny_B_Actl1 : Outport  Port=2
  Ford_LaHandsOff_B_Actl1 : Outport  Port=3
  Ford_LsmcBrkDecelEnbl_D_Rq1 : Outport  Port=4
  Ford_LsmcBrk_Tq_Rq : Outport  Port=5
  Ford_TjaHandsOnCnfdnc_B_Est1 : Outport  Port=6
  Ford_TrlrAn_An_TrgtCalc : Outport  Port=7

== system Ford_T3T6_ArchCnctnDigrm/Ford CFs/FIH Read and Write/FIH Initialize/CF061A_FordBlaBoxInitAndFctCall1 ==
  EcuId : Inport
  FordActvNiblCtrlEnad : Inport  Port=2
  FordEpsSysSt : Inport  Port=3
  FordLaneDprtrWarnEnad : Inport  Port=4
  FordLaneKeepingAssiEnad : Inport  Port=5
  FordPullDriftCmpEnad : Inport  Port=6
  FordTrlrBackupAssiEnad : Inport  Port=7
  ActvNiblCtrlFctCallSts : Outport
  FordLaneKeepingAssiFctCallSts : Outport  Port=2
  LaneDprtrWarnFctCallSts : Outport  Port=3
  LatCtrlFctCallSts : Outport  Port=4
  PullDriftCmpFctCallSts : Outport  Port=5

== system Ford_T3T6_ArchCnctnDigrm/Ford CFs/FIH Read and Write/FIH Initialize/CF093A_FordBlaBoxInitAndFctCall2 ==
  EcuId : Inport
  FordEpsSysSt : Inport  Port=2
  FordEvasSteerAssiEna : Inport  Port=3
  SteerTqDstbcRejctnEna : Inport  Port=4
  EvasSteerAssiFctCallSts : Outport
  SteerTqDstbcRejctnFctCallSts : Outport  Port=2

== system Ford_T3T6_ArchCnctnDigrm/Ford CFs/FIH Read and Write/FIH Read/CF053A_FordBlaBoxEpsRead ==
  ActvParkAssiTqFild : Inport
  AppldFinalMotTq : Inport  Port=2
  BoostCrvAssiTq : Inport  Port=3
  BoostCrvInpTq : Inport  Port=4
  EcuId : Inport  Port=5
  EngTqClass : Inport  Port=6
  ExtAgCtrlSpdVld : Inport  Port=7
  ExtAgCtrlSteerPinionAgVelVld : Inport  Port=8
  FildVehSpd : Inport  Port=9
  FordCmpdHwPosn : Inport  Port=10
  FordCmpdHwPosnQlyFac : Inport  Port=11
  FordEpsSysSt : Inport  Port=12
  FordMaxAsscTq : Inport  Port=13
  FordRelHwPosn : Inport  Port=14
  FordVehTireCircum : Inport  Port=15
  HwVel : Inport  Port=16
  INTAgCtrlStat1 : Inport  Port=17
  InpTqRaw : Inport  Port=18
  RackToPinionRat : Inport  Port=19
  ReqdFinalMotTq : Inport  Port=20
  SelctvDrvgModSteerMod : Inport  Port=21
  SemiAutParlParkAgCtrlSts1 : Inport  Port=22
  SemiAutParlParkAgCtrlSts2 : Inport  Port=23
  SemiAutParlParkAgCtrlSts3 : Inport  Port=24
  SemiAutParlParkAgCtrlSts4 : Inport  Port=25
  SemiAutParlParkAgCtrlSts5 : Inport  Port=26
  SemiAutParlParkAgCtrlSts6 : Inport  Port=27
  VehSpd : Inport  Port=28
  VehSteerRat : Inport  Port=29
  VehWhlBas : Inport  Port=30
  ExtAgCtrlStsInt : Inport  Port=31
  GetRefTmr100MicroSec32bit : Inport  Port=32
  FIH_Read_APA_Torque_Filtered : Outport
  FIH_Read_AngleControlState : Outport  Port=2
  FIH_Read_EACSpeedValid : Outport  Port=3
  FIH_Read_EAC_SPAVelocityValid : Outport  Port=4
  FIH_Read_EPS_Assist_Torque : Outport  Port=5
  FIH_Read_EPS_ColumnVelocity : Outport  Port=6
  FIH_Read_EPS_CompSPA_QF : Outport  Port=7
  FIH_Read_EPS_Final_Motor_Tq_App : Outport  Port=8
  FIH_Read_EPS_Final_Motor_Tq_Rq : Outport  Port=9
  FIH_Read_EPS_InputTorqueFilt : Outport  Port=10
  FIH_Read_EPS_InputTorqueRaw : Outport  Port=11
  FIH_Read_EPS_Personalization : Outport  Port=12
  FIH_Read_EPS_Rel_SteeringAngle : Outport  Port=13
  FIH_Read_EPS_SteeringAngle : Outport  Port=14
  FIH_Read_EPS_System_Time : Outport  Port=15
  FIH_Read_EPS_TireCircumference : Outport  Port=16
  FIH_Read_EPS_VehicleSpeed : Outport  Port=17
  FIH_Read_EPS_VehicleSpeed_Raw : Outport  Port=18
  FIH_Read_EngineSize : Outport  Port=19
  FIH_Read_MaxAssistanceTorque : Outport  Port=20
  FIH_Read_RackPinionRatio : Outport  Port=21
  FIH_Read_SAPPAngleControlStat1 : Outport  Port=22
  FIH_Read_SAPPAngleControlStat2 : Outport  Port=23
  FIH_Read_SAPPAngleControlStat3 : Outport  Port=24
  FIH_Read_SAPPAngleControlStat4 : Outport  Port=25
  FIH_Read_SAPPAngleControlStat5 : Outport  Port=26
  FIH_Read_SteMdule_D_Stat : Outport  Port=27
  FIH_Read_VehicleSteeringRatio : Outport  Port=28
  FIH_Read_WheelBase : Outport  Port=29
  FIH_Read_TBA_EAC_Status : Outport  Port=30

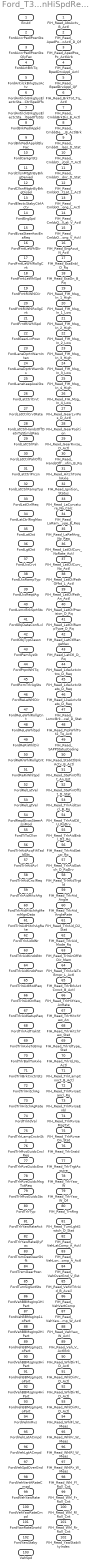
== system Ford_T3T6_ArchCnctnDigrm/Ford CFs/FIH Read and Write/FIH Read/CF054A_FordBlaBoxCanHiSpdRead ==
  EcuId : Inport
  FordAccrPedlPosnSts : Inport  Port=2
  FordAccrPedlPosnStsQlyFac : Inport  Port=3
  FordActBrkTq : Inport  Port=4
  FordAntilckBrkgSysActv : Inport  Port=5
  FordAntilckBrkgSysElectcStabyCtrlSpaOffs : Inport  Port=6
  FordAntilckBrkgSysElectcStabyCtrlSpaOffsSts : Inport  Port=7
  FordBrkPedlAppld : Inport  Port=8
  FordBrkPedlAppldQlyFac : Inport  Port=9
  FordCanIgnSts : Inport  Port=10
  FordCllsnMtgtnByBrkgDenied : Inport  Port=11
  FordCllsnMtgtnByBrkgDisad : Inport  Port=12
  FordElectcStabyCtrlActv : Inport  Port=13
  FordEngSpd : Inport  Port=14
  FordEvasSteerAssiEnaReq : Inport  Port=15
  FordFrntLeWhlDir : Inport  Port=16
  FordFrntLeWhlRollgCnt : Inport  Port=17
  FordFrntLeWhlSpd : Inport  Port=18
  FordFrntRiWhlDir : Inport  Port=19
  FordFrntRiWhlRollgCnt : Inport  Port=20
  FordFrntRiWhlSpd : Inport  Port=21
  FordGearLvrPosn : Inport  Port=22
  FordLaneDprtrWarnInten : Inport  Port=23
  FordLaneDprtrWarnSts : Inport  Port=24
  FordLaneKeepAssiSts : Inport  Port=25
  FordLatCtrlCrvt : Inport  Port=26
  FordLatCtrlCrvtRate : Inport  Port=27
  FordLatCtrlHandsOffDetnTqStimlsReq : Inport  Port=28
  FordLatCtrlPah : Inport  Port=29
  FordLatCtrlPahOffs : Inport  Port=30
  FordLatCtrlPrcsn : Inport  Port=31
  FordLatCtrlRampTyp : Inport  Port=32
  FordLatCtrlReq : Inport  Port=33
  FordLatCtrlRngMax : Inport  Port=34
  FordLatDst : Inport  Port=35
  FordLgtDst : Inport  Port=36
  FordLksCrvt : Inport  Port=37
  FordLksRampTyp : Inport  Port=38
  FordLksReqdAg : Inport  Port=39
  FordLsmcBrkSprtSts : Inport  Port=40
  FordObjDataConfLvl : Inport  Port=41
  FordObjTypClassn : Inport  Port=42
  FordPamSysSt : Inport  Port=43
  FordPrpnWhlTq : Inport  Port=44
  FordRcmTrlrAgSts : Inport  Port=45
  FordReLeWhlDir : Inport  Port=46
  FordReLeWhlRollgCnt : Inport  Port=47
  FordReLeWhlSpd : Inport  Port=48
  FordReRiWhlDir : Inport  Port=49
  FordReRiWhlRollgCnt : Inport  Port=50
  FordReRiWhlSpd : Inport  Port=51
  FordRelLatVel : Inport  Port=52
  FordRelLgtVel : Inport  Port=53
  FordReqdEvasSteerAssiMod : Inport  Port=54
  FordTiToCllsn : Inport  Port=55
  FordTrlrAidAcqFihTadIdSts : Inport  Port=56
  FordTrlrAidAvl : Inport  Port=57
  FordTrlrAidCnclReq : Inport  Port=58
  FordTrlrAidHitchAg : Inport  Port=59
  FordTrlrAidHitchAgMemMgnData : Inport  Port=60
  FordTrlrAidHitchAgRate : Inport  Port=61
  FordTrlrAidIdNr : Inport  Port=62
  FordTrlrAidKnobBtn : Inport  Port=63
  FordTrlrAidKnobPosn : Inport  Port=64
  FordTrlrAidModReq : Inport  Port=65
  FordTrlrAidOnReq : Inport  Port=66
  FordTrlrAidSetupReq : Inport  Port=67
  FordTrlrAidTrakSt : Inport  Port=68
  FordTrlrAxleToBmp : Inport  Port=69
  FordTrlrBallToAxle : Inport  Port=70
  FordTrlrBrkCnctnSts : Inport  Port=71
  FordTrlrHitchAg : Inport  Port=72
  FordTrlrHitchAgRate : Inport  Port=73
  FordTrlrIdVal : Inport  Port=74
  FordTrlrLampCnctnSts : Inport  Port=75
  FordTrlrRvsGuidcCnclReq : Inport  Port=76
  FordTrlrRvsGuidcEna : Inport  Port=77
  FordTrlrRvsGuidcMsgTxtReq : Inport  Port=78
  FordTrlrRvsGuidcSts : Inport  Port=79
  FordTrlrTyp : Inport  Port=80
  FordTrlrYawRateAct : Inport  Port=81
  FordTrlrYawRateQlyFac : Inport  Port=82
  FordTrsmDesGearShift : Inport  Port=83
  FordTrsmGearPosn : Inport  Port=84
  FordTurnSigSwtSts : Inport  Port=85
  FordVehBBMsgInp1HiPart : Inport  Port=86
  FordVehBBMsgInp1LoPart : Inport  Port=87
  FordVehBBMsgInp2HiPart : Inport  Port=88
  FordVehBBMsgInp2LoPart : Inport  Port=89
  FordVehBBMsgInp3HiPart : Inport  Port=90
  FordVehBBMsgInp3LoPart : Inport  Port=91
  FordVehBBMsgInp4HiPart : Inport  Port=92
  FordVehBBMsgInp4LoPart : Inport  Port=93
  FordVehInRvs : Inport  Port=94
  FordVehLatACmpd : Inport  Port=95
  FordVehLgtACmpd : Inport  Port=96
  FordVehSpdOverGnd : Inport  Port=97
  FordVehVertARateCmpd : Inport  Port=98
  FordVehYawRate : Inport  Port=99
  FordVehYawRateCmpd : Inport  Port=100
  FordYawRateSnsrId : Inport  Port=101
  FordYawStaby : Inport  Port=102
  VehSpd : Inport  Port=103
  FIH_Read_AbsActv_B_Actl : Outport
  FIH_Read_ApedPosPcActl_D_Qf : Outport  Port=2
  FIH_Read_ApedPos_Pc_ActlArb : Outport  Port=3
  FIH_Read_BpedDrvAppl_Actl : Outport  Port=4
  FIH_Read_BpedDrvAppl_QF : Outport  Port=5
  FIH_Read_BrkTot_Tq_Actl : Outport  Port=6
  FIH_Read_CmbbBrkDis_B_Actl : Outport  Port=7
  FIH_Read_CmbbDeny_B_ActlBrk : Outport  Port=8
  FIH_Read_CmbbObjClass_D_Stat : Outport  Port=9
  FIH_Read_CmbbObjColl_T_Actl : Outport  Port=10
  FIH_Read_CmbbObjConfdnc_D_Stat : Outport  Port=11
  FIH_Read_CmbbObjDistLat_L_Actl : Outport  Port=12
  FIH_Read_CmbbObjDistLong_L_Actl : Outport  Port=13
  FIH_Read_CmbbObjRelLat_V_Actl : Outport  Port=14
  FIH_Read_CmbbObjRelLong_V_Actl : Outport  Port=15
  FIH_Read_EngAout_N_Actl : Outport  Port=16
  FIH_Read_EsaEnbl_D_Rq : Outport  Port=17
  FIH_Read_EsaOn_B_Rq : Outport  Port=18
  FIH_Read_FIH_Msg_In_1_High : Outport  Port=19
  FIH_Read_FIH_Msg_In_1_Low : Outport  Port=20
  FIH_Read_FIH_Msg_In_2_High : Outport  Port=21
  FIH_Read_FIH_Msg_In_2_Low : Outport  Port=22
  FIH_Read_FIH_Msg_In_3_High : Outport  Port=23
  FIH_Read_FIH_Msg_In_3_Low : Outport  Port=24
  FIH_Read_FIH_Msg_In_4_High : Outport  Port=25
  FIH_Read_FIH_Msg_In_4_Low : Outport  Port=26
  FIH_Read_GearLvrPos_D_Actl : Outport  Port=27
  FIH_Read_GearPosition : Outport  Port=28
  FIH_Read_GearRvrse_D_Actl : Outport  Port=29
  FIH_Read_HandsOffCnfm_B_Rq : Outport  Port=30
  FIH_Read_HitchToVehAxle : Outport  Port=31
  FIH_Read_Ignition_Status : Outport  Port=32
  FIH_Read_LaCurvature_No_Calc : Outport  Port=33
  FIH_Read_LaRampType_B_Req : Outport  Port=34
  FIH_Read_LaRefAng_No_Req : Outport  Port=35
  FIH_Read_LatCtlCurv_NoRate_Actl : Outport  Port=36
  FIH_Read_LatCtlCurv_No_Actl : Outport  Port=37
  FIH_Read_LatCtlPathOffst_L_Actl : Outport  Port=38
  FIH_Read_LatCtlPath_An_Actl : Outport  Port=39
  FIH_Read_LatCtlPrecision_D_Rq : Outport  Port=40
  FIH_Read_LatCtlRampType_D_Rq : Outport  Port=41
  FIH_Read_LatCtlRangeMax : Outport  Port=42
  FIH_Read_LatCtl_D_Rq : Outport  Port=43
  FIH_Read_LdwActvIntns_D_Req : Outport  Port=44
  FIH_Read_LdwActvStats_D_Req : Outport  Port=45
  FIH_Read_LkaActvStats_D_Req : Outport  Port=46
  FIH_Read_LsmcBrkDecel_D_Stat : Outport  Port=47
  FIH_Read_PrplWhlTot2_Tq_Actl : Outport  Port=48
  FIH_Read_SAPPStatusCoding : Outport  Port=49
  FIH_Read_StabCtlBrkActv_B_Actl : Outport  Port=50
  FIH_Read_StePinOffst_An_Est : Outport  Port=51
  FIH_Read_StePinOffst_D_Stat : Outport  Port=52
  FIH_Read_TrlrAidCancl_B_Rq : Outport  Port=53
  FIH_Read_TrlrAidCtl_U_RqDrv : Outport  Port=54
  FIH_Read_TrlrAidEnbl_D2_Rq : Outport  Port=55
  FIH_Read_TrlrAidSetup_Rq : Outport  Port=56
  FIH_Read_TrlrAidSwtch_D_RqDrv : Outport  Port=57
  FIH_Read_TrlrAidTrgtId : Outport  Port=58
  FIH_Read_TrlrAid_Angle : Outport  Port=59
  FIH_Read_TrlrAid_AngleRate : Outport  Port=60
  FIH_Read_TrlrAid_D2_Stat : Outport  Port=61
  FIH_Read_TrlrAid_Mode_Rq : Outport  Port=62
  FIH_Read_TrlrAnOffstDir_Mem : Outport  Port=63
  FIH_Read_TrlrAxleToBmpr_L_Actl : Outport  Port=64
  FIH_Read_TrlrBrkActCnnct_B_Actl : Outport  Port=65
  FIH_Read_TrlrHitYaw_AnRate : Outport  Port=66
  FIH_Read_TrlrHitchYaw_An : Outport  Port=67
  FIH_Read_TrlrHitchYaw_Stat : Outport  Port=68
  FIH_Read_TrlrIdType_Stat : Outport  Port=69
  FIH_Read_TrlrId_No_Actl : Outport  Port=70
  FIH_Read_TrlrLampCnnct_B_Actl : Outport  Port=71
  FIH_Read_TrlrRvrseCancl_Rq : Outport  Port=72
  FIH_Read_TrlrRvrseEnbl : Outport  Port=73
  FIH_Read_TrlrRvrseMsgTxt : Outport  Port=74
  FIH_Read_TrlrRvrseOn_Stat : Outport  Port=75
  FIH_Read_TrlrSnsId : Outport  Port=76
  FIH_Read_TrlrTrgtAcquire : Outport  Port=77
  FIH_Read_TrlrYaw_W : Outport  Port=78
  FIH_Read_TrlrYaw_W_Qf : Outport  Port=79
  FIH_Read_TrnRng : Outport  Port=80
  FIH_Read_TurnLghtSwtch_D_Stat : Outport  Port=81
  FIH_Read_VehLatComp_A_Actl : Outport  Port=82
  FIH_Read_VehLongComp_A_Actl : Outport  Port=83
  FIH_Read_VehOverGnd_V_Est : Outport  Port=84
  FIH_Read_VehVTrlrAid_B_Avail : Outport  Port=85
  FIH_Read_VehVertComp : Outport  Port=86
  FIH_Read_VehYawComp_W_Actl : Outport  Port=87
  FIH_Read_VehYaw_W_Actl : Outport  Port=88
  FIH_Read_Veh_V_ActlBrk : Outport  Port=89
  FIH_Read_WhlDirFl_D_Actl : Outport  Port=90
  FIH_Read_WhlDirFr_D_Actl : Outport  Port=91
  FIH_Read_WhlDirRl_D_Actl : Outport  Port=92
  FIH_Read_WhlDirRr_D_Actl : Outport  Port=93
  FIH_Read_WhlFl_W_Meas : Outport  Port=94
  FIH_Read_WhlFr_W_Meas : Outport  Port=95
  FIH_Read_WhlRl_W_Meas : Outport  Port=96
  FIH_Read_WhlRr_W_Meas : Outport  Port=97
  FIH_Read_Whl_Fl_Roll_Cnt : Outport  Port=98
  FIH_Read_Whl_Fr_Roll_Cnt : Outport  Port=99
  FIH_Read_Whl_Rl_Roll_Cnt : Outport  Port=100
  FIH_Read_Whl_Rr_Roll_Cnt : Outport  Port=101
  FIH_Read_YawStabilityIndex : Outport  Port=102

== system Ford_T3T6_ArchCnctnDigrm/Ford CFs/FIH Read and Write/FIH Read/CF056A_FordBlaBoxVldRead ==
  APedlPosVld : Inport
  AbsActvVld : Inport  Port=2
  AppldFinalMotTqVld : Inport  Port=3
  BrkTqArbnVld : Inport  Port=4
  BrkTqDrvVld : Inport  Port=5
  BrkTqVld : Inport  Port=6
  EcuId : Inport  Port=7
  EngRPMVld : Inport  Port=8
  EsaAbsVld : Inport  Port=9
  EsaIpcVld : Inport  Port=10
  EsaIpmAVld : Inport  Port=11
  EscActvVld : Inport  Port=12
  FihMsgInp1Vld : Inport  Port=13
  FihMsgInp2Vld : Inport  Port=14
  FihMsgInp3Vld : Inport  Port=15
  FihMsgInp4Vld : Inport  Port=16
  FrntLeWhlCntDirVld : Inport  Port=17
  FrntLeWhlSpdVld : Inport  Port=18
  FrntRiWhlCntDirVld : Inport  Port=19
  FrntRiWhlSpdVld : Inport  Port=20
  GearLvrPosVld : Inport  Port=21
  IgnStsVld : Inport  Port=22
  InpTqRawVld : Inport  Port=23
  LATCTLIpmAVld : Inport  Port=24
  LSMCBrkSprtVld : Inport  Port=25
  LaIpmAVld : Inport  Port=26
  LatAVld : Inport  Port=27
  LongAVld : Inport  Port=28
  PamStsVld : Inport  Port=29
  ParkAidMsgVld : Inport  Port=30
  ParkAidSnsrVld : Inport  Port=31
  PropTqVld : Inport  Port=32
  ReLeWhlCntDirVld : Inport  Port=33
  ReLeWhlSpdVld : Inport  Port=34
  ReRiWhlCntDirVld : Inport  Port=35
  ReRiWhlSpdVld : Inport  Port=36
  RelSpaVld : Inport  Port=37
  RvsGearVld : Inport  Port=38
  SdmChassisVld : Inport  Port=39
  SpaOffsVld : Inport  Port=40
  SpaVelVld : Inport  Port=41
  TrlrBackupAssiAvlVld : Inport  Port=42
  TrlrBackupAssiCnclReqVld : Inport  Port=43
  TrlrBackupAssiEnaVld : Inport  Port=44
  TrlrBackupAssiHitchAgVld : Inport  Port=45
  TrlrBackupAssiHitchRateVld : Inport  Port=46
  TrlrBackupAssiKnobPosnVld : Inport  Port=47
  TrlrBackupAssiKnobVld : Inport  Port=48
  TrlrBackupAssiMeasurmentVld : Inport  Port=49
  TrlrBackupAssiModReqVld : Inport  Port=50
  TrlrBackupAssiRvsVld : Inport  Port=51
  TrlrBackupAssiTarVld : Inport  Port=52
  TrlrBackupAssiTrackStVld : Inport  Port=53
  TrlrBackupAssiYawRateVld : Inport  Port=54
  TrlrBrkCnctnVld : Inport  Port=55
  TrlrLampCnctnVld : Inport  Port=56
  TrlrTarOffsVld : Inport  Port=57
  TrlrTarToBmpVld : Inport  Port=58
  TurnSigVld : Inport  Port=59
  VehSpdOverGndVld : Inport  Port=60
  VehSpdVld : Inport  Port=61
  YawRateRawVld : Inport  Port=62
  YawRateVld : Inport  Port=63
  YawStabyVld : Inport  Port=64
  FordVehBrkPedlVld : Inport  Port=65
  VertAccelValid : Inport  Port=66
  FilteredVehicleSpeedValid : Inport  Port=67
  FIH_Read_Signal_Status : Outport
  FIH_Read_Signal_Status2 : Outport  Port=2
  FIH_Read_Signal_Status_PassThru : Outport  Port=3

== system Ford_T3T6_ArchCnctnDigrm/Ford CFs/FIH Read and Write/FIH Read/CF057A_FordBlaBoxDiagcRead ==
  ANCDiagcStsInt : Inport
  ANCIntSts : Inport  Port=2
  BPRActvnCntInt : Inport  Port=3
  ESAIntSts : Inport  Port=4
  EcuId : Inport  Port=5
  LATCTLIntSts : Inport  Port=6
  LDWDiagcStsInt : Inport  Port=7
  LDWIntSts : Inport  Port=8
  LKAIntSts : Inport  Port=9
  PDCIntSts : Inport  Port=10
  STDRIntSts : Inport  Port=11
  SrvPDCRstValInt : Inport  Port=12
  TBAIntSts : Inport  Port=13
  TSCActvnCntInt : Inport  Port=14
  FIH_Read_ANC_Ext_Diag_Status : Outport
  FIH_Read_ANC_Int_Status_DID : Outport  Port=2
  FIH_Read_BPR_Activation_Cnt : Outport  Port=3
  FIH_Read_ESA_Int_Status_DID : Outport  Port=4
  FIH_Read_LATCTL_Int_Status_DID : Outport  Port=5
  FIH_Read_LDW_Ext_Diag_Status : Outport  Port=6
  FIH_Read_LDW_Int_Status_DID : Outport  Port=7
  FIH_Read_LKA_Int_Status_DID : Outport  Port=8
  FIH_Read_PDC_Int_Status_DID : Outport  Port=9
  FIH_Read_PDC_Service_DID : Outport  Port=10
  FIH_Read_STDR_Int_Status_DID : Outport  Port=11
  FIH_Read_TBA_Int_Status_DID : Outport  Port=12
  FIH_Read_TSC_Activation_Cnt : Outport  Port=13

== system Ford_T3T6_ArchCnctnDigrm/Ford CFs/FIH Read and Write/FIH Read/CF059A_FordBlaBoxFeatStRead ==
  EcuId : Inport
  FordActvNiblCtrlArbiterCmd : Inport  Port=2
  FordActvNiblCtrlEnad : Inport  Port=3
  FordBrkPlsRejctnEnad : Inport  Port=4
  FordEvasSteerAssiArbiterCmd : Inport  Port=5
  FordEvasSteerAssiEnad : Inport  Port=6
  FordLaneCenteringAssiEnad : Inport  Port=7
  FordLaneDprtrWarnArbiterCmd : Inport  Port=8
  FordLaneDprtrWarnEnad : Inport  Port=9
  FordLaneKeepingAssiArbiterCmd : Inport  Port=10
  FordLaneKeepingAssiEnad : Inport  Port=11
  FordLatCtrlArbiterCmd : Inport  Port=12
  FordPullDriftCmpArbiterCmd : Inport  Port=13
  FordPullDriftCmpEnad : Inport  Port=14
  FordPullDriftCmpLrngArbiterCmd : Inport  Port=15
  FordResrchFctEnad : Inport  Port=16
  FordSteerTqDstbcRejctnArbiterCmd : Inport  Port=17
  FordTqSteerCmpEnad : Inport  Port=18
  FordTrfcJamAssiEnad : Inport  Port=19
  FordTrlrBackupAssi5WhlEnad : Inport  Port=20
  FordTrlrBackupAssiEnad : Inport  Port=21
  FordTrlrBackupAssiTRGEnad : Inport  Port=22
  FIH_Read_ANC_Arbiter : Outport
  FIH_Read_ESA_Arbiter : Outport  Port=2
  FIH_Read_FIH_EoL_Config : Outport  Port=3
  FIH_Read_LATCTL_Arbiter : Outport  Port=4
  FIH_Read_LDW_Arbiter : Outport  Port=5
  FIH_Read_LKA_Arbiter : Outport  Port=6
  FIH_Read_PDCLearning_Arbiter : Outport  Port=7
  FIH_Read_PDC_Arbiter : Outport  Port=8
  FIH_Read_STDR_Arbiter : Outport  Port=9

== system Ford_T3T6_ArchCnctnDigrm/Ford CFs/FIH Read and Write/FIH Read/CF062A_FordBlaBoxNvmRead ==
  EcuId : Inport
  FordBlaBoxActvNiblCtrlByte : Inport  Port=2
  FordBlaBoxLaneAssiByte : Inport  Port=3
  FordBlaBoxPullDriftCmpByte : Inport  Port=4
  FordBlaBoxTrlrBackupByte : Inport  Port=5
  FIH_ANC_Read_NV_Byte : Outport
  FIH_LA_Read_NV_Byte : Outport  Port=2
  FIH_PDC_Read_NV_Byte : Outport  Port=3
  FIH_TBA_Read_NV_Byte : Outport  Port=4
